simulink model "SocModel"  (R2024a)
settings: Solver=FixedStepDiscrete  StartTime=0.0  StopTime=1  FixedStep=0.2  RelTol=1e-3
undefined symbols (not defined in the file or in its folder): capacityAh, dt, SOC
settings Model: Creator=sudhakars2  LastModifiedBy=mgmsu
settings OptimizationCC: DefaultParameterBehavior=Inlined  EnhancedBackFolding=on  PassReuseOutputArgsAs=Individual arguments  ZeroExternalMemoryAtStartup=off  ZeroInternalMemoryAtStartup=off  OptimizeBlockOrder=speed  DifferentSizesBufferReuse=on  OptimizationCustomize=off  EfficientTunableParamExpr=on
settings DebuggingCC: ParameterTunabilityLossMsg=error
settings HardwareCC: ProdBitPerLong=64  ProdHWDeviceType=Intel->x86-64 (Linux 64)
settings SFSimCC: SimGenImportedTypeDefs=on  MATLABDynamicMemAlloc=off  SimTargetLang=C++
settings RTWCC: Description=AUTOSAR Adaptive  SystemTargetFile=autosar_adaptive.tlc  HardwareBoard=Embedded Coder Linux Docker Container  GenCodeOnly=on  TemplateMakefile=ert_default_tmf  Toolchain=AUTOSAR Adaptive Linux Executable  DataTypeReplacement=CDataTypesFixedWidth  TargetLang=C++
settings CodeAppCC: ForceParamTrailComments=on  IgnoreCustomStorageClasses=off  MaxIdLength=63  OperatorAnnotations=on  SimulinkDataObjDesc=on  SFDataObjDesc=on  InsertBlockDesc=on
settings AUTOSARAdaptiveTargetCC: TargetFcnLib=ansi_tfl_table_tmw.mat  GenFloatMathFcnCalls=NOT IN USE  TargetLangStandard=C++11 (ISO)  CodeReplacementLibrary=C++ Standard Library Mutex  UtilityFuncGeneration=Auto  MultiwordTypeDef=System defined  MultiwordLength=2048  DynamicStringBufferSize=256  GenerateFullHeader=on  InferredTypesCompatibility=off  GenerateSampleERTMain=off  GenerateTestInterfaces=off  ModelReferenceCompliant=on  ParMdlRefBuildCompliant=on  CompOptLevelCompliant=on  ConcurrentExecutionCompliant=on  IncludeMdlTerminateFcn=on  CombineOutputUpdateFcns=on  CombineSignalStateStructs=off  GroupInternalDataByFunction=off  SuppressErrorStatus=on  IncludeFileDelimiter=Auto  ERTCustomFileBanners=off  SupportAbsoluteTime=on  LogVarNameModifier=rt_  MatFileLogging=off  CodeInterfacePackaging=C++ class  PurelyIntegerCode=off  SupportNonFinite=off  SupportComplex=on  SupportContinuousTime=off  SupportNonInlinedSFcns=off  RemoveDisableFunc=off  RemoveResetFunc=on  SupportVariableSizeSignals=off  ParenthesesLevel=Nominal  CastingMode=Nominal  MATLABClassNameForMDSCustomization=Simulink.SoftwareTarget.TargetSpecificTriggerConfigurationBase  ModelStepFunctionPrototypeControlCompliant=off  CPPClassGenCompliant=on  AutosarCompliant=on  MDXCompliant=off  GRTInterface=off  GenerateAllocFcn=off  UseToolchainInfoCompliant=on  GenerateSharedConstants=on  CoderGroups=[]  AccessMethods=[]  LookupTableObjectStructAxisOrder=2,1,3,4,...  LUTObjectStructOrderExplicitValues=Size,Breakpoints,Table  LUTObjectStructOrderEvenSpacing=Size,Table,Breakpoints  ArrayLayout=Column-major  UnsupportedSFcnMsg=error  ERTHeaderFileRootName=$R$E  ERTSourceFileRootName=$R$E  ERTDataFileRootName=$R_data  InstructionSetFMA=off  OptimizeReductions=off  LogToMDFFile=off  DSAsUniqueAccess=off  ExtMode=off  ExtModeTransport=0  ExtModeStaticAlloc=on  ExtModeAutomaticAllocSize=on  ExtModeMaxTrigDuration=1000  ExtModeStaticAllocSize=1000000  ExtModeTesting=off  ExtModeMexFile=ext_xcp  ExtModeIntrfLevel=Level2 - Open  InlinedParameterPlacement=NonHierarchical  TargetOS=BareBoardExample  MultiInstanceErrorCode=Error  RootIOFormat=Structure reference  RTWCAPISignals=off  RTWCAPIParams=off  RTWCAPIStates=off  RTWCAPIRootIO=off  ERTSrcFileBannerTemplate=ert_code_template.cgt  ERTHdrFileBannerTemplate=ert_code_template.cgt  ERTDataSrcFileTemplate=ert_code_template.cgt  ERTDataHdrFileTemplate=ert_code_template.cgt  ERTCustomFileTemplate=example_file_process.tlc  EnableDataOwnership=off  SignalDisplayLevel=10  ParamTuneLevel=10  GlobalDataDefinition=Auto  DataDefinitionFile=global.c  GlobalDataReference=Auto  ERTFilePackagingFormat=Modular  RateTransitionBlockCode=Inline  DataReferenceFile=global.h  PreserveExpressionOrder=off  PreserveIfCondition=off  ConvertIfToSwitch=on  PreserveExternInFcnDecls=on  PreserveStaticInFcnDecls=on  SuppressUnreachableDefaultCases=on  EnableSignedLeftShifts=on  EnableSignedRightShifts=on  ImplementImageWithCVMat=off  IndentStyle=K&R  IndentSize=2  NewlineStyle=Default  MaxLineWidth=80  EnableUserReplacementTypes=off  MaxIdInt64=INT64_MAX  MinIdInt64=INT64_MIN  MaxIdUint64=UINT64_MAX  MaxIdInt32=INT32_MAX  MinIdInt32=INT32_MIN  MaxIdUint32=UINT32_MAX  MaxIdInt16=INT16_MAX  MinIdInt16=INT16_MIN  MaxIdUint16=UINT16_MAX  MaxIdInt8=INT8_MAX  MinIdInt8=INT8_MIN  MaxIdUint8=UINT8_MAX  BooleanTrueId=true  BooleanFalseId=false  MemSecPackage=--- None ---  MemSecDataConstants=Default  MemSecDataIO=Default  MemSecDataInternal=Default  MemSecDataParameters=Default  MemSecFuncInitTerm=Default  MemSecFuncExecute=Default  MemSecFuncSharedUtil=Default  GroupConstants=Default  GroupRootInputs=Default  GroupRootOutputs=Default  GroupInternal=Default  GroupParameters=Default  GroupDataTransfer=Default  GroupSharedLocalDataStores=Default  GroupInstanceSpecificParameters=Default  GroupModelData=Default  ArrayContainerType=std::array  AutosarSchemaVersion=00049  AutosarMaxShortNameLength=128  AdaptiveAutosarXCPServerTransportLayer=XCPOnTCPIP  AdaptiveAutosarXCPServerTCPIPAddress=10.30.85.189  AdaptiveAutosarXCPServerPort=22255  AdaptiveAutosarXCPServerVerbosity=off  AdaptiveAutosarUseCustomXCPServer=off
settings ConfigComp: CovBoundaryAbsTol=1.0e-5

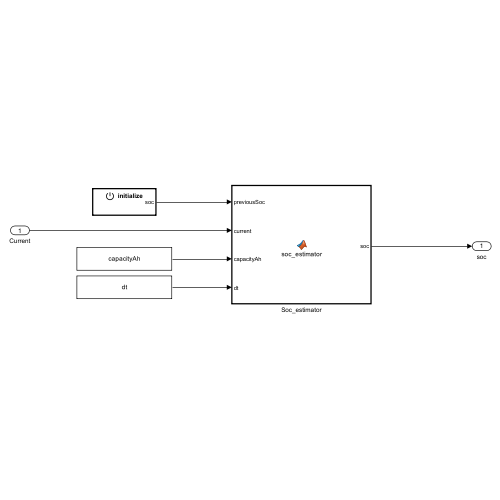
[thumbnail: Simulink's stored preview of the top-level diagram]
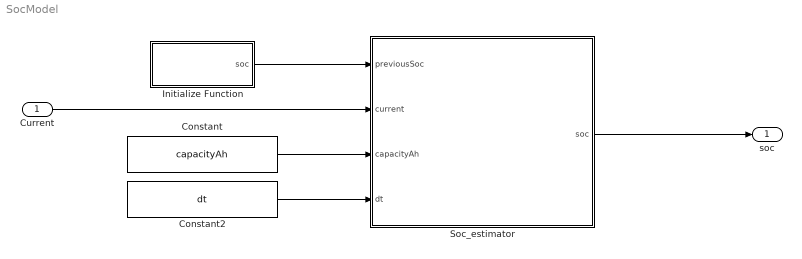
== system SocModel ==
  Current : Inport
  Constant : Constant  Value=capacityAh
  Constant2 : Constant  Value=dt
  Initialize Function : Subsystem  TreatAsAtomicUnit=on
  Soc_estimator : MATLAB Function  TreatAsAtomicUnit=on
  soc : Outport
  wires:
  Current/1 -> Soc_estimator/2(current)
  Constant/1 -> Soc_estimator/3(capacityAh)
  Constant2/1 -> Soc_estimator/4(dt)
  Soc_estimator/1(soc) -> soc/1
  Initialize Function/1(soc) -> Soc_estimator/1(previousSoc)

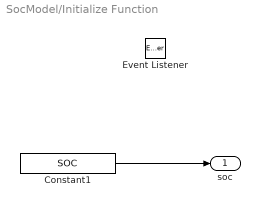
== system SocModel/Initialize Function ==
  Constant1 : Constant  Value=SOC
  Event Listener : EventListener  DisableCoverage=on  EventName=reset
  soc : Outport
  wires:
  Constant1/1 -> soc/1

== matlab function SocModel/Soc_estimator ==
  data: previousSoc input; soc output; current input; capacityAh input; dt input
function soc = soc_estimator(previousSoc,...
                             current,...
                             capacityAh,...
                             dt)

capacityAs = capacityAh * 3600;

deltaSoc = (current * dt / capacityAs) * 100;

soc = previousSoc - deltaSoc;

soc = max(0,min(100,soc)); 

end
